simulink model "RLC_dynamic_system"  (R2024a)
settings: Solver=FixedStepDiscrete  StartTime=0.0  StopTime=10.0  RelTol=1e-3
settings Model: Creator=VICTUS  LastModifiedBy=VICTUS

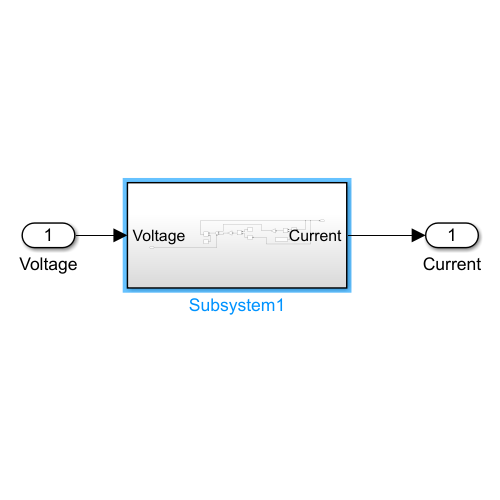
[thumbnail: Simulink's stored preview of the top-level diagram]
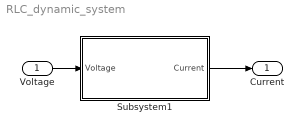
== system RLC_dynamic_system ==
  Voltage : Inport
  Subsystem1 : Subsystem
  Current : Outport
  wires:
  Voltage/1 -> Subsystem1/1(Voltage)
  Subsystem1/1(Current) -> Current/1

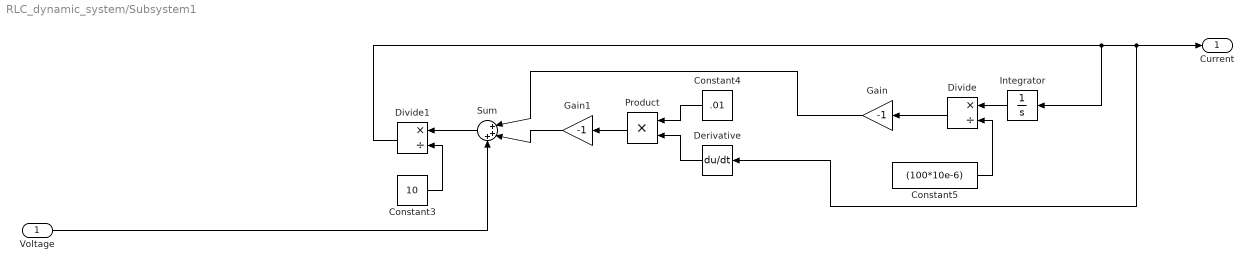
== system RLC_dynamic_system/Subsystem1 ==
  Voltage : Inport
  Constant3 : Constant  Value=10
  Constant4 : Constant  Value=.01
  Constant5 : Constant  Value=(100*10e-6)
  Derivative : Derivative
  Divide : Product  Inputs=*/
  Divide1 : Product  Inputs=*/
  Gain : Gain  Gain=-1
  Gain1 : Gain  Gain=-1
  Integrator : Integrator
  Product : Product
  Sum : Sum  Inputs=|+++
  Current : Outport
  wires:
  Divide1/1 -> Integrator/1, Current/1, Derivative/1
  Divide/1 -> Gain/1
  Constant5/1 -> Divide/2
  Integrator/1 -> Divide/1
  Sum/1 -> Divide1/1
  Gain/1 -> Sum/1
  Constant3/1 -> Divide1/2
  Constant4/1 -> Product/1
  Voltage/1 -> Sum/3
  Derivative/1 -> Product/2
  Product/1 -> Gain1/1
  Gain1/1 -> Sum/2
